simulink model "DDMR2"  (R2015a)
settings: Solver=ode3  StartTime=0.0  StopTime=22  FixedStep=0.02  RelTol=1e-3
settings Model: Creator=PinkWink  LastModifiedBy=MrJohd
settings DataIOCC: SignalLoggingSaveFormat=ModelDataLogs
settings OptimizationCC: ExpressionDepthLimit=2147483647
settings DebuggingCC: UnderspecifiedInitializationDetection=Classic  MergeDetectMultiDrivingBlocksExec=none  SolverPrmCheckMsg=warning  FcnCallInpInsideContextMsg=UseLocalSettings  StateNameClashWarn=warning
settings GRTTargetCC: CombineOutputUpdateFcns=off  GRTInterface=on

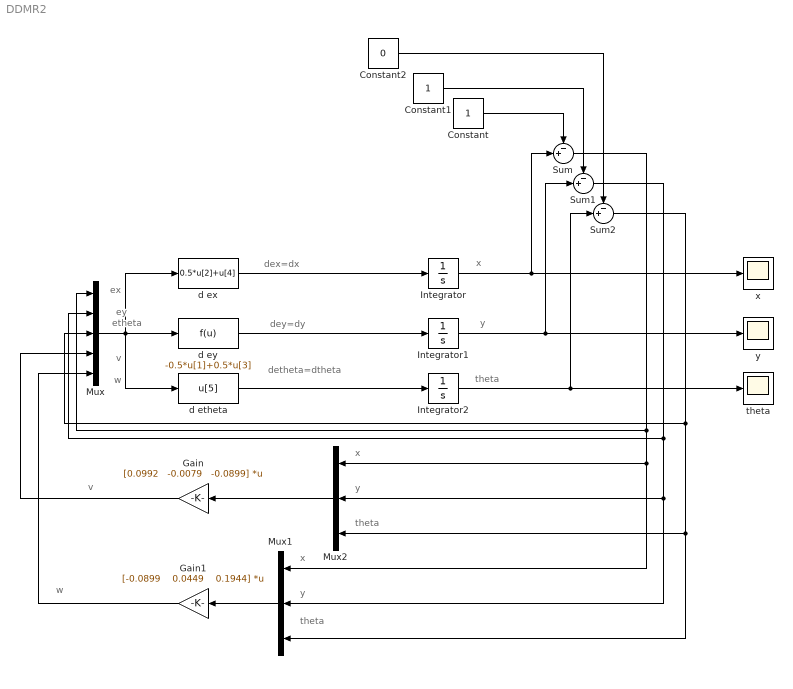
== system DDMR2 ==
  note: detheta=dtheta
  note: dey=dy
  note: dex=dx
  note: w
  note: v
  note: etheta
  note: ey
  note: ex
  note: w
  note: v
  note: x
  note: theta
  note: y
  note: x
  note: y
  note: theta
  note: x
  note: y
  note: theta
  Constant : Constant
  Constant1 : Constant
  Constant2 : Constant  Value=0
  Gain : Gain  Gain="[0.0992   -0.0079   -0.0899]"  Multiplication=Matrix(K*u)
  Gain1 : Gain  Gain="[-0.0899    0.0449    0.1944]"  Multiplication=Matrix(K*u)
  Integrator : Integrator
  Integrator1 : Integrator
  Integrator2 : Integrator
  Mux : Mux  Inputs=5
  Mux1 : Mux  Inputs=3
  Mux2 : Mux  Inputs=3
  Sum : Sum  Inputs=-+|
  Sum1 : Sum  Inputs=-+|
  Sum2 : Sum  Inputs=-+|
  d etheta : Fcn  Expr=u[5]
  d ex : Fcn  Expr=0.5*u[2]+u[4]
  d ey : Fcn  Expr=-0.5*u[1]+0.5*u[3]
  theta : Scope
  x : Scope
      settings: YMin=0.72  YMax=0.9  SaveName=ScopeData3
  y : Scope
      settings: YMin=0.72  YMax=0.9
  wires:
  Mux/1 -> d ey/1, d ex/1, d etheta/1
  Mux2/1 -> Gain/1
  Constant/1 -> Sum/1
  Sum1/1 -> Mux/2, Mux1/2, Mux2/2
  Sum2/1 -> Mux/3, Mux1/3, Mux2/3
  d ex/1 -> Integrator/1
  d etheta/1 -> Integrator2/1
  Mux1/1 -> Gain1/1
  d ey/1 -> Integrator1/1
  Integrator/1 -> Sum/2, x/1
  Integrator1/1 -> Sum1/2, y/1
  Integrator2/1 -> Sum2/2, theta/1
  Constant1/1 -> Sum1/1
  Constant2/1 -> Sum2/1
  Gain/1 -> Mux/4
  Gain1/1 -> Mux/5
  Sum/1 -> Mux/1, Mux1/1, Mux2/1
